simulink model "invertedPendolum"  (R2019b)
settings: Solver=VariableStepAuto  StartTime=0.0  StopTime=60  FixedStep=0.0001  RelTol=1e-4
InitFcn:
  | simulationVar
values from neighbouring files (symbols this model uses):
  tauMotMax = Ka * Id    (= 6208417600)    [simulationVar.m]
undefined symbols (not defined in the file or in its folder): smiData, X, Y, Z
libraries: sm_lib x768, simulink x6, nesl_utility x3
(part 13 of 13)

== system invertedPendolum/Interfaccia grafica/coperchio_1/UNI_5739_M5_x_405_RIGID ==
  ReferenceFrame : sm_lib/Frames and Transforms/Reference Frame
  Solid : sm_lib/Body Elements/File Solid  ExtGeomFileName=UNI 5739 M5 x 40_ipt_708e3c23.STEP  UnitType=FromFile  ExtGeomFileUnits=m  StepReaderType=HEX  ExportEntireGeometry=off  InertiaType=Custom  Mass=smiData.Solid(7).mass  MassUnits=kg  CenterOfMass=smiData.Solid(7).CoM  CenterOfMassUnits=mm  MomentsOfInertia=smiData.Solid(7).MoI  MomentsOfInertiaUnits=kg*mm^2  ProductsOfInertia=smiData.Solid(7).PoI  ProductsOfInertiaUnits=kg*mm^2  BasedOnType=DensityFromFile  Density=1000  DensityUnits=kg/m^3  DoExposeReferenceFrame=on  SerializedFrames=<Frames/>  GraphicType=FromGeometry  MarkerShape=Sphere  MarkerSize=10  GraphicVisPropType=SimpleVisualProperties  GraphicDiffuseColor=smiData.Solid(7).color  GraphicSpecularColor=[0.5 0.5 0.5 1.0]  GraphicAmbientColor=[0.15 0.15 0.15 1.0]  GraphicEmissiveColor=[0.0 0.0 0.0 1.0]  GraphicShininess=75  GraphicOpacity=smiData.Solid(7).opacity
  Transform : sm_lib/Frames and Transforms/Rigid Transform  TranslationMethod=Cartesian  TranslationStandardOffset=0  TranslationLengthUnit=mm  TranslationStandardAxis=+Z  TranslationCartesianOffset=smiData.RigidTransform(44).translation  TranslationROffset=0  TranslationROffsetUnits=m  TranslationZOffset=0  TranslationZOffsetUnits=m  TranslationThetaOffset=0  TranslationThetaOffsetUnits=deg  RotationMethod=ArbitraryAxis  RotationAngleUnits=rad  RotationStandardAxis=+Z  RotationAngle=smiData.RigidTransform(44).angle  RotationArbitraryAxis=smiData.RigidTransform(44).axis  FollAlignAxisA=+X  BaseAlignAxisA=+Y  FollAlignAxisB=+Y  BaseAlignAxisB=+Z  RotationSequenceAxes=FollowerAxes  RotationSequence=XYX  RotationSequenceAngles=[0 0 0]  RotationSequenceAnglesUnits=deg  RotationMatrix=[1 0 0; 0 1 0; 0 0 1]
  F : PMIOPort  Side=Left
  connections:
  Transform/RConn1 -- F/RConn1
  Transform/LConn1 -- ReferenceFrame/RConn1 -- Solid/RConn1

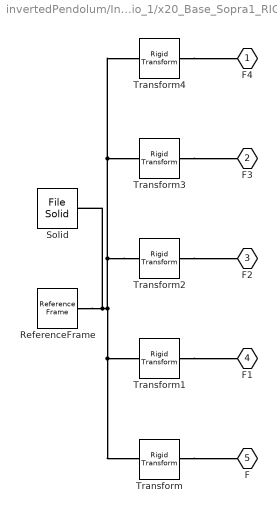
== system invertedPendolum/Interfaccia grafica/coperchio_1/x20_Base_Sopra1_RIGID ==
  ReferenceFrame : sm_lib/Frames and Transforms/Reference Frame
  Solid : sm_lib/Body Elements/File Solid  ExtGeomFileName=20_Base_Sopra_ipt_abe47da0.STEP  UnitType=FromFile  ExtGeomFileUnits=m  StepReaderType=HEX  ExportEntireGeometry=off  InertiaType=Custom  Mass=smiData.Solid(2).mass  MassUnits=kg  CenterOfMass=smiData.Solid(2).CoM  CenterOfMassUnits=mm  MomentsOfInertia=smiData.Solid(2).MoI  MomentsOfInertiaUnits=kg*mm^2  ProductsOfInertia=smiData.Solid(2).PoI  ProductsOfInertiaUnits=kg*mm^2  BasedOnType=DensityFromFile  Density=1000  DensityUnits=kg/m^3  DoExposeReferenceFrame=on  SerializedFrames=<Frames/>  GraphicType=FromGeometry  MarkerShape=Sphere  MarkerSize=10  GraphicVisPropType=SimpleVisualProperties  GraphicDiffuseColor=smiData.Solid(2).color  GraphicSpecularColor=[0.5 0.5 0.5 1.0]  GraphicAmbientColor=[0.15 0.15 0.15 1.0]  GraphicEmissiveColor=[0.0 0.0 0.0 1.0]  GraphicShininess=75  GraphicOpacity=smiData.Solid(2).opacity
  Transform : sm_lib/Frames and Transforms/Rigid Transform  TranslationMethod=Cartesian  TranslationStandardOffset=0  TranslationLengthUnit=mm  TranslationStandardAxis=+Z  TranslationCartesianOffset=smiData.RigidTransform(6).translation  TranslationROffset=0  TranslationROffsetUnits=m  TranslationZOffset=0  TranslationZOffsetUnits=m  TranslationThetaOffset=0  TranslationThetaOffsetUnits=deg  RotationMethod=ArbitraryAxis  RotationAngleUnits=rad  RotationStandardAxis=+Z  RotationAngle=smiData.RigidTransform(6).angle  RotationArbitraryAxis=smiData.RigidTransform(6).axis  FollAlignAxisA=+X  BaseAlignAxisA=+Y  FollAlignAxisB=+Y  BaseAlignAxisB=+Z  RotationSequenceAxes=FollowerAxes  RotationSequence=XYX  RotationSequenceAngles=[0 0 0]  RotationSequenceAnglesUnits=deg  RotationMatrix=[1 0 0; 0 1 0; 0 0 1]
  Transform1 : sm_lib/Frames and Transforms/Rigid Transform  TranslationMethod=Cartesian  TranslationStandardOffset=0  TranslationLengthUnit=mm  TranslationStandardAxis=+Z  TranslationCartesianOffset=smiData.RigidTransform(42).translation  TranslationROffset=0  TranslationROffsetUnits=m  TranslationZOffset=0  TranslationZOffsetUnits=m  TranslationThetaOffset=0  TranslationThetaOffsetUnits=deg  RotationMethod=ArbitraryAxis  RotationAngleUnits=rad  RotationStandardAxis=+Z  RotationAngle=smiData.RigidTransform(42).angle  RotationArbitraryAxis=smiData.RigidTransform(42).axis  FollAlignAxisA=+X  BaseAlignAxisA=+Y  FollAlignAxisB=+Y  BaseAlignAxisB=+Z  RotationSequenceAxes=FollowerAxes  RotationSequence=XYX  RotationSequenceAngles=[0 0 0]  RotationSequenceAnglesUnits=deg  RotationMatrix=[1 0 0; 0 1 0; 0 0 1]
  Transform2 : sm_lib/Frames and Transforms/Rigid Transform  TranslationMethod=Cartesian  TranslationStandardOffset=0  TranslationLengthUnit=mm  TranslationStandardAxis=+Z  TranslationCartesianOffset=smiData.RigidTransform(62).translation  TranslationROffset=0  TranslationROffsetUnits=m  TranslationZOffset=0  TranslationZOffsetUnits=m  TranslationThetaOffset=0  TranslationThetaOffsetUnits=deg  RotationMethod=ArbitraryAxis  RotationAngleUnits=rad  RotationStandardAxis=+Z  RotationAngle=smiData.RigidTransform(62).angle  RotationArbitraryAxis=smiData.RigidTransform(62).axis  FollAlignAxisA=+X  BaseAlignAxisA=+Y  FollAlignAxisB=+Y  BaseAlignAxisB=+Z  RotationSequenceAxes=FollowerAxes  RotationSequence=XYX  RotationSequenceAngles=[0 0 0]  RotationSequenceAnglesUnits=deg  RotationMatrix=[1 0 0; 0 1 0; 0 0 1]
  Transform3 : sm_lib/Frames and Transforms/Rigid Transform  TranslationMethod=Cartesian  TranslationStandardOffset=0  TranslationLengthUnit=mm  TranslationStandardAxis=+Z  TranslationCartesianOffset=smiData.RigidTransform(64).translation  TranslationROffset=0  TranslationROffsetUnits=m  TranslationZOffset=0  TranslationZOffsetUnits=m  TranslationThetaOffset=0  TranslationThetaOffsetUnits=deg  RotationMethod=ArbitraryAxis  RotationAngleUnits=rad  RotationStandardAxis=+Z  RotationAngle=smiData.RigidTransform(64).angle  RotationArbitraryAxis=smiData.RigidTransform(64).axis  FollAlignAxisA=+X  BaseAlignAxisA=+Y  FollAlignAxisB=+Y  BaseAlignAxisB=+Z  RotationSequenceAxes=FollowerAxes  RotationSequence=XYX  RotationSequenceAngles=[0 0 0]  RotationSequenceAnglesUnits=deg  RotationMatrix=[1 0 0; 0 1 0; 0 0 1]
  Transform4 : sm_lib/Frames and Transforms/Rigid Transform  TranslationMethod=Cartesian  TranslationStandardOffset=0  TranslationLengthUnit=mm  TranslationStandardAxis=+Z  TranslationCartesianOffset=smiData.RigidTransform(66).translation  TranslationROffset=0  TranslationROffsetUnits=m  TranslationZOffset=0  TranslationZOffsetUnits=m  TranslationThetaOffset=0  TranslationThetaOffsetUnits=deg  RotationMethod=ArbitraryAxis  RotationAngleUnits=rad  RotationStandardAxis=+Z  RotationAngle=smiData.RigidTransform(66).angle  RotationArbitraryAxis=smiData.RigidTransform(66).axis  FollAlignAxisA=+X  BaseAlignAxisA=+Y  FollAlignAxisB=+Y  BaseAlignAxisB=+Z  RotationSequenceAxes=FollowerAxes  RotationSequence=XYX  RotationSequenceAngles=[0 0 0]  RotationSequenceAnglesUnits=deg  RotationMatrix=[1 0 0; 0 1 0; 0 0 1]
  F4 : PMIOPort  Side=Left
  F3 : PMIOPort  Port=2  Side=Right
  F2 : PMIOPort  Port=3  Side=Left
  F1 : PMIOPort  Port=4  Side=Right
  F : PMIOPort  Port=5  Side=Left
  connections:
  Transform4/RConn1 -- F4/RConn1
  Transform3/RConn1 -- F3/RConn1
  Transform2/RConn1 -- F2/RConn1
  Transform1/RConn1 -- F1/RConn1
  Transform/RConn1 -- F/RConn1
  Transform2/LConn1 -- Transform4/LConn1 -- Transform3/LConn1 -- Transform1/LConn1 -- Transform/LConn1 -- ReferenceFrame/RConn1 -- Solid/RConn1

== matlab function invertedPendolum/Reverse Pendolum/system ==
  data: x input; xdot output size=4; u input; y output; brake input
function [xdot,y] = pendoloNotLinSys(x,u,brake)
%PENDOLONOTLINSYS Summary of this function goes here
% xDot1:= q2 acc    [rad/s^2]
% xDot2:= q2 vel    [rad/s]
% xDot3:= q1 acc    [rad/s^2]
% xDot4:= q1 vel    [rad/s]

% x1:= q2 dot    [rad/s]
% x2:= q2        [rad]
% x3:= q1 dot    [rad/s]
% x4:= q1        [rad]

% u:= Coppia motore [g/s^2 * mm]
% brake:= true change D2 and shutdown u

coder.extrinsic('evalin', 'assignin')

D1 = 0;                  % Needed in order to set variable class correctly
D1 = evalin('base','D1'); % Read value from workspace

Id = 0;                  % Needed in order to set variable class correctly
Id = evalin('base','Id'); % Read value from workspace

Ibtot = 0;                  % Needed in order to set variable class correctly
Ibtot = evalin('base','Ibtot'); % Read value from workspace

Kmgl = 0;                  % Needed in order to set variable class correctly
Kmgl = evalin('base','Kmgl'); % Read value from workspace

tauMotMax = 0;
tauMotMax = evalin('base','tauMotMax'); % Read value from workspace

rhoInd = 0;                  % Needed in order to set variable class correctly
rhoInd = evalin('base','rhoInd'); % Read value from workspace

rhoMec = 0;                  % Needed in order to set variable class correctly
rhoMec = evalin('base','rhoMec'); % Read value from workspace

D2 = 0;                  % Needed in order to set variable class correctly
D2 = evalin('base','D2'); % Read value from workspace

attDyn = 0;                  % Needed in order to set variable class correctly
attDyn = evalin('base','attDyn'); % Read value from workspace


% Calcoli notevoli:
% fprintf('Kmgl= %f, Ibtot=%f\t', Kmgl, Ibtot); 
skmgl = (Kmgl/Ibtot)*sin(x(4));
% fprintf('skmgl= %f\t', skmgl); 
d1friz = (D1*x(3))/Ibtot;
% fprintf('d1friz= %f\t', d1friz); 
% d2x1 = D2*x(1);
% D2 è in funzione di u, v e si ottiene moltiplicando per l'inerzia i dati
% sperimentali
duty=abs(u/tauMotMax);
if(abs(x(1))>0.001)
%     d2x1 = (((rhoInd)*abs(u/tauMotMax)+ rhoMec)*x(1) + sign(x(1))*attDyn)*Id;
    d2x1 = ((rhoInd+rhoMec)*x(1))*Id + sign(x(1))*attDyn;
%     d2x1 = ((rhoInd*duty+rhoMec)*x(1))*Id + sign(x(1))*attDyn;

else
    d2x1 = 0;

end
% fprintf('d2x1= %f\tduty=%f\n', d2x1,duty); 

xdot=zeros(4,1);
xdot(1) = -(1/Ibtot+1/Id)*d2x1 - skmgl + d1friz + (1/Ibtot+1/Id)*u;
xdot(2) = x(1);
xdot(3) = d2x1/Ibtot + skmgl - d1friz - u/Ibtot;
% fprintf('xdot(3)= %f\n', xdot(3));  
xdot(4) = x(3);


%per ora supponiamo di poter osservare tutto il sistema
y=x;

end

== matlab function invertedPendolum/Reverse Pendolum/saturation ==
  data: x input; xSat output; reset output
function [xSat,reset]  = phisicReaction(x)
%PHISICREACTION Summary of this function goes here
% Funzione che letto lo stato, in caso di urto con la base cambia
% in maniera realistica lo stato introducendo una saturazione.

% xDot1:= q2 acc    [rad/s^2]
% xDot2:= q2 vel    [rad/s]
% xDot3:= q1 acc    [rad/s^2]
% xDot4:= q1 vel    [rad/s]

% x1:= q2 dot    [rad/s]
% x2:= q2        [rad]
% x3:= q1 dot    [rad/s]
% x4:= q1        [rad]

coder.extrinsic('evalin', 'assignin')
q1Max = 0;                  % Needed in order to set variable class correctly
q1Max = evalin('base','q1Max'); % Read value from workspace

xSat=x;
if((abs(x(4))>q1Max)&&(sign(x(3))==sign(x(4))))
    xSat(3)=-x(3)*0.1;          % dissipazione di energia
    xSat(4)=sign(x(4))*(q1Max*0.99999);   % riposizionamento
    
    %to reset integrator state
    assignin('base','x0',xSat); % Assign value back to workspace
    reset=1;
else
    reset=0;
end

end

== matlab function invertedPendolum/Reverse Pendolum/x0Loader ==
  data: x0 output
function x0 = loadX0()
% xDot1:= q2 acc    [rad/s^2]
% xDot2:= q2 vel    [rad/s]
% xDot3:= q1 acc    [rad/s^2]
% xDot4:= q1 vel    [rad/s]

% x1:= q2 dot    [rad/s]
% x2:= q2        [rad]
% x3:= q1 dot    [rad/s]
% x4:= q1        [rad]
coder.extrinsic('evalin', 'assignin')
x0 = zeros(4,1);          % Needed in order to set variable class correctly
x0 = evalin('base','x0'); % Read value from workspace

== matlab function invertedPendolum/Reverse Pendolum/x0Loader1 ==
  data: x0 output
function x0 = loadX0()
% xDot1:= q2 acc    [rad/s^2]
% xDot2:= q2 vel    [rad/s]
% xDot3:= q1 acc    [rad/s^2]
% xDot4:= q1 vel    [rad/s]

% x1:= q2 dot    [rad/s]
% x2:= q2        [rad]
% x3:= q1 dot    [rad/s]
% x4:= q1        [rad]
coder.extrinsic('evalin', 'assignin')
x0 = zeros(4,1);          % Needed in order to set variable class correctly
x0 = evalin('base','x0'); % Read value from workspace

== matlab function invertedPendolum/MATLAB Function ==
  data: mTotDes input; x input; tauMot output size=1
function tauMot = Mwant(mTotDes, x)
% x1:= q2 dot    [rad/s]
% x2:= q2        [rad]
% x3:= q1 dot    [rad/s]
% x4:= q1        [rad]
% tauMot:= Coppia motore [g/s^2 * mm]

coder.extrinsic('evalin', 'assignin')
Kmgl = 0;                  % Needed in order to set variable class correctly
Kmgl = evalin('base','Kmgl'); % Read value from workspace

D1 = 0;                  % Needed in order to set variable class correctly
D1 = evalin('base','D1'); % Read value from workspace

% D2 = 0;                  % Needed in order to set variable class correctly
% D2 = evalin('base','D2'); % Read value from workspace

tauMotMax = 0;           % Needed in order to set variable class correctly
tauMotMax = evalin('base','tauMotMax'); % Read value from workspace

Id = 0;                  % Needed in order to set variable class correctly
Id = evalin('base','Id'); % Read value from workspace


rhoInd = 0;                  % Needed in order to set variable class correctly
rhoInd = evalin('base','rhoInd'); % Read value from workspace

rhoMec = 0;                  % Needed in order to set variable class correctly
rhoMec = evalin('base','rhoMec'); % Read value from workspace

attDyn = 0;                  % Needed in order to set variable class correctly
attDyn = evalin('base','attDyn'); % Read value from workspace

% Frenata del motore in funzione della velocità
% d2x1 = (((rhoInd) *abs(u/tauMotMax) + rhoMec)*x(1) + sign(x(1))*uDym)*Id;

% d2x1 = (((rhoInd) + rhoMec)*x(1) + sign(x(1))*uDym)*Id;
% duty=abs(u/tauMotMax);
if(abs(x(1))>0.001)
%     d2x1 = (((rhoInd)*abs(u/tauMotMax)+ rhoMec)*x(1) + sign(x(1))*attDyn)*Id;
    d2x1 = ((rhoInd+rhoMec)*x(1))*Id + sign(x(1))*attDyn;
%     d2x1 = ((rhoInd*duty+rhoMec)*x(1))*Id + sign(x(1))*attDyn;

else
    d2x1 = 0;

end

% fprintf("d2x1=%f\n",d2x1);

tauMot = -mTotDes + d2x1 + Kmgl*sin(x(4)) - D1*x(3);
% fprintf("tauMot=%f\n",tauMot);
end
